simulink model "control_structure_a"  (R2015a)
settings: Solver=ode45  StartTime=0.0  StopTime=t_stop  MaxStep=0.01  MinStep=0.001  RelTol=1e-3
values from neighbouring files (symbols this model uses):
  A_dA = 0.3    [ex1.m]    (also in ex2.m = 0.01; ex3.m = 0)
  A_dT = 0    [ex1.m]    (also in ex2.m; ex3.m)
  A_dY = 0    [ex1.m]    (also in ex2.m = 0.1; ex3.m)
  A_r = 0.1    [ex1.m]    (also in ex2.m = 0; ex3.m = 3)
  input_switch = 1    [ex1.m]    (also in ex2.m = -1; ex3.m)
  switch_dT = 0    [ex1.m]    (also in ex3.m = 1)
  switch_dY = 1    [ex1.m]    (also in ex2.m = -1; ex3.m)
  w_dT = 0    [ex1.m]    (also in ex3.m)
  w_dY = 0    [ex1.m]    (also in ex3.m)
libraries: cstblocks x2, simulink x1
settings Model: Creator=Riccardo  LastModifiedBy=Riccardo

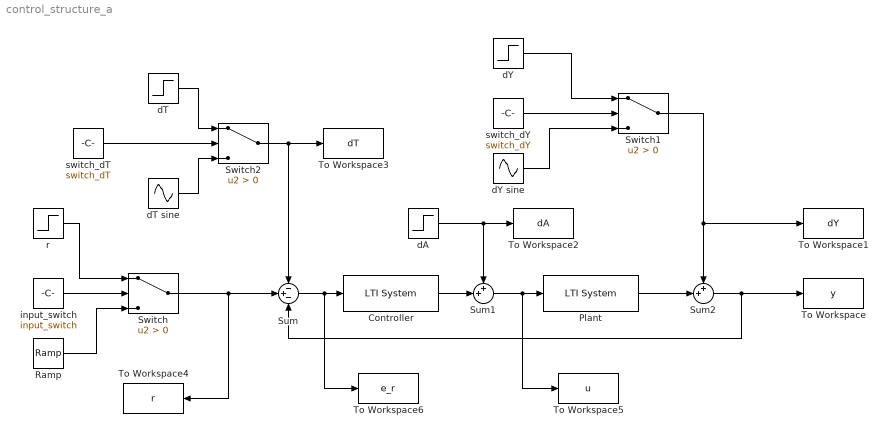
== system control_structure_a ==
  Controller : cstblocks/LTI System  sys=C  IC=[]
  Plant : cstblocks/LTI System  sys=G  IC=[]
  Ramp : simulink/Sources/Ramp  slope=A_r  start=0  X0=0
  Sum : Sum  Inputs=-+-
  Sum1 : Sum  Inputs=++|
  Sum2 : Sum  Inputs=++|
  Switch : Switch  Criteria=u2 > Threshold
  Switch1 : Switch  Criteria=u2 > Threshold
  Switch2 : Switch  Criteria=u2 > Threshold
  To Workspace : ToWorkspace  VariableName=y  SaveFormat=Structure With Time  SampleTime=-1
  To Workspace1 : ToWorkspace  VariableName=dY  SaveFormat=Structure With Time  SampleTime=-1
  To Workspace2 : ToWorkspace  VariableName=dA  SaveFormat=Structure With Time  SampleTime=-1
  To Workspace3 : ToWorkspace  VariableName=dT  SaveFormat=Structure With Time  SampleTime=-1
  To Workspace4 : ToWorkspace  VariableName=r  SaveFormat=Structure With Time  SampleTime=-1
  To Workspace5 : ToWorkspace  VariableName=u  SaveFormat=Structure With Time  SampleTime=-1
  To Workspace6 : ToWorkspace  VariableName=e_r  SaveFormat=Structure With Time  SampleTime=-1
  "dA " : Step  Time=0  After=A_dA  SampleTime=0
  "dT " : Step  Time=0  After=A_dT  SampleTime=0
  "dT sine " : Sin  Amplitude=A_dT  Frequency=w_dT  SampleTime=0
  dY : Step  Time=0  After=A_dY  SampleTime=0
  dY sine : Sin  Amplitude=A_dY  Frequency=w_dY  SampleTime=0
  "input_switch " : Constant  Value=input_switch
  "r " : Step  Time=0  After=A_r  SampleTime=0
  switch_dT : Constant  Value=switch_dT
  switch_dY : Constant  Value=switch_dY
  wires:
  Sum/1 -> To Workspace6/1, Controller/1
  "dA "/1 -> To Workspace2/1, Sum1/1
  Sum1/1 -> To Workspace5/1, Plant/1
  Controller/1 -> Sum1/2
  Plant/1 -> Sum2/2
  Sum2/1 -> Sum/3, To Workspace/1
  Switch/1 -> Sum/2, To Workspace4/1
  "input_switch "/1 -> Switch/2
  "r "/1 -> Switch/1
  Ramp/1 -> Switch/3
  Switch1/1 -> To Workspace1/1, Sum2/1
  dY/1 -> Switch1/1
  dY sine/1 -> Switch1/3
  switch_dY/1 -> Switch1/2
  "dT "/1 -> Switch2/1
  Switch2/1 -> To Workspace3/1, Sum/1
  switch_dT/1 -> Switch2/2
  "dT sine "/1 -> Switch2/3
